simulink model "chap7_5sim"  (Simulink 8.1)
settings: Solver=ode4  StartTime=0.0  StopTime=10  RelTol=1e-3
settings Model: Creator=eleliuj  LastModifiedBy=liujk  ExtModeTrigMode=oneshot  ExtModeArmWhenConnect=off
settings DataIOCC: Decimation=100  LimitDataPoints=off  SaveOutput=off  SaveTime=off  SignalLoggingName=sigsOut
settings OptimizationCC: BooleanDataType=off  InitFltsAndDblsToZero=on
settings DebuggingCC: SaveWithParameterizedLinksMsg=none  SignalResolutionControl=TryResolveAllWithWarning  SolverPrmCheckMsg=none  MultiTaskDSMMsg=warning  MultiTaskCondExecSysMsg=none  StrictBusMsg=None
settings HardwareCC: TargetUnknown=on
settings RTWCC: IncludeERTFirstTime=on

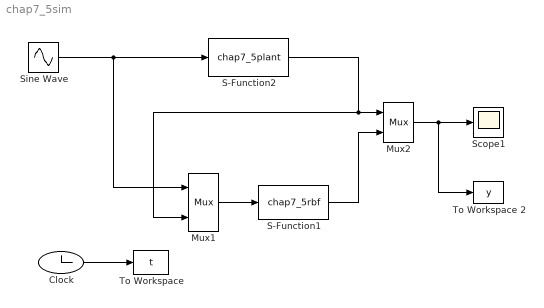
== system chap7_5sim ==
  Clock : Clock
  Mux1 : Mux  Inputs=2
  Mux2 : Mux  Inputs=2
  S-Function1 : S-Function  FunctionName=chap7_5rbf  EnableBusSupport=off
  S-Function2 : S-Function  FunctionName=chap7_5plant  EnableBusSupport=off
  Scope1 : Scope
      settings: TimeRange=0.2  YMin=-0.25  YMax=3  MaxDataPoints=50000  SampleInput=on  SampleTime=0.001
  Sine Wave : Sin  SampleTime=0
  To Workspace : ToWorkspace  VariableName=t  SampleTime=-1
  To Workspace 2 : ToWorkspace  VariableName=y  SampleTime=-1
  wires:
  Mux1/1 -> S-Function1/1
  S-Function2/1 -> Mux1/2, Mux2/1
  Sine Wave/1 -> S-Function2/1, Mux1/1
  S-Function1/1 -> Mux2/2
  Clock/1 -> To Workspace/1
  Mux2/1 -> Scope1/1, To Workspace 2/1
